simulink model "full_order_as_tf_with_controller_to_pdf"  (R2015b)
settings: Solver=VariableStepAuto  StartTime=0.0  StopTime=10.0  RelTol=1e-3
undefined symbols (not defined in the file): Iq, J_pro, Kt, Kv, R, TS
libraries: simulink x1
settings Model: Creator=Morten  LastModifiedBy=Morten

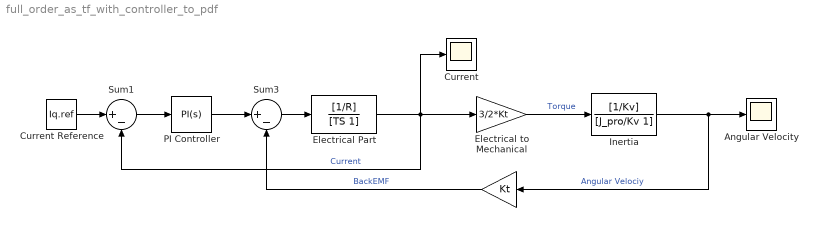
== system full_order_as_tf_with_controller_to_pdf ==
  "             " : Gain  Gain=Kt
  "Angular Velocity " : Scope
  Current Reference : Constant  Value=Iq.ref
  "Current " : Scope
  "Electrical Part " : TransferFcn  Numerator=[1/R]  Denominator=[TS 1]
  "Electrical to Mechanical " : Gain  Gain=3/2*Kt
  "Inertia " : TransferFcn  Numerator=[1/Kv]  Denominator=[J_pro/Kv 1]
  "PI Controller " : simulink/Continuous/PID Controller  Controller=PI  TimeDomain=Continuous-time  SampleTime=-1  IntegratorMethod=Forward Euler  FilterMethod=Forward Euler  Form=Parallel  UseFilter=on  ControllerParametersSource=internal  P=0.0157  I=2.5637  D=0  N=100  InitialConditionSource=internal  InitialConditionForIntegrator=0  InitialConditionForFilter=0  ExternalReset=none  LimitOutput=off  UpperSaturationLimit=inf  LowerSaturationLimit=-inf  LinearizeAsGain=on  AntiWindupMode=none  Kb=1  TrackingMode=off  Kt=1  PParamMin=[]  PParamMax=[]  IParamMin=[]  IParamMax=[]  DParamMin=[]  DParamMax=[]  NParamMin=[]  NParamMax=[]  KbParamMin=[]  KbParamMax=[]  KtParamMin=[]  KtParamMax=[]  POutMin=[]  POutMax=[]  IOutMin=[]  IOutMax=[]  DOutMin=[]  DOutMax=[]  NOutMin=[]  NOutMax=[]  KbOutMin=[]  KbOutMax=[]  KtOutMin=[]  KtOutMax=[]  IntegratorOutMin=[]  IntegratorOutMax=[]  FilterOutMin=[]  FilterOutMax=[]  SumOutMin=[]  SumOutMax=[]  SumI1OutMin=[]  SumI1OutMax=[]  SumI2OutMin=[]  SumI2OutMax=[]  SumI3OutMin=[]  SumI3OutMax=[]  SumDOutMin=[]  SumDOutMax=[]  SaturationOutMin=[]  SaturationOutMax=[]  IntegratorContinuousStateAttributes=''  IntegratorStateMustResolveToSignalObject=off  IntegratorRTWStateStorageClass=Auto  FilterContinuousStateAttributes=''  FilterStateMustResolveToSignalObject=off  FilterRTWStateStorageClass=Auto  DifferentiatorICPrevScaledInput=0  DifferentiatorOutMin=[]  DifferentiatorOutMax=[]
  Sum1 : Sum  Inputs=|+-
  Sum3 : Sum  Inputs=|+-
  wires:
  "             "/1 -> Sum3/2  "BackEMF"
  Sum3/1 -> "Electrical Part "/1
  "Electrical Part "/1 -> Sum1/2, "Current "/1, "Electrical to Mechanical "/1  "Current"
  "Electrical to Mechanical "/1 -> "Inertia "/1  "Torque"
  "Inertia "/1 -> "Angular Velocity "/1, "             "/1  "Angular Velociy"
  Current Reference/1 -> Sum1/1
  Sum1/1 -> "PI Controller "/1
  "PI Controller "/1 -> Sum3/1
